simulink model "optical_flow_sim"  (R2024b)
settings: Solver=VariableStepAuto  StartTime=0.0  StopTime=30  RelTol=1e-3
undefined symbols (not defined in the file or in its folder): twist
libraries: ros2lib x4
settings Model: Creator=DCHOME  LastModifiedBy=DCHOME

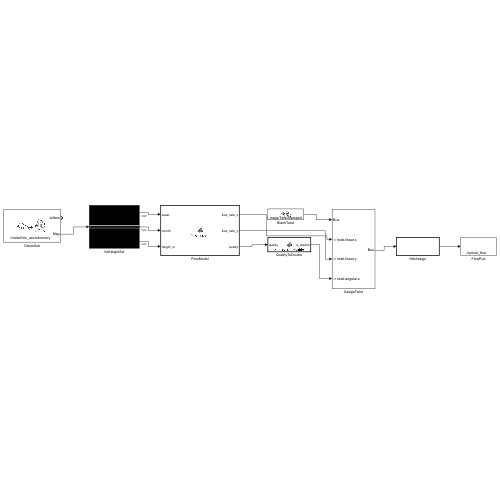
[thumbnail: Simulink's stored preview of the top-level diagram]
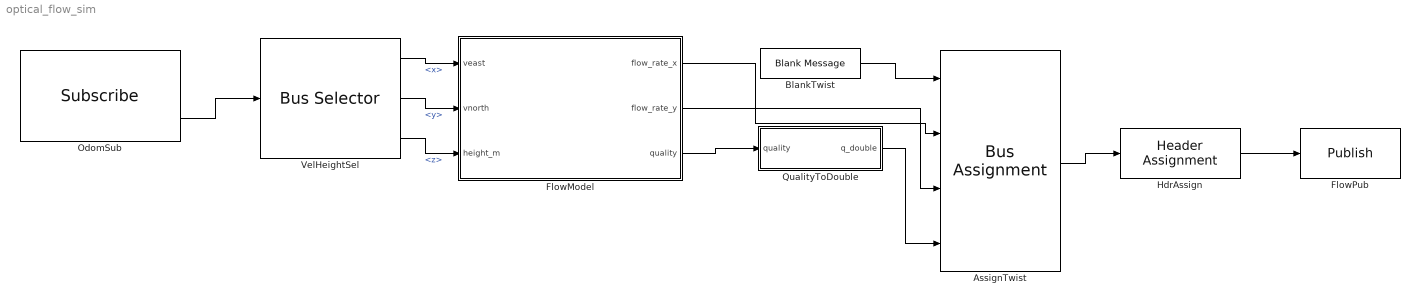
== system optical_flow_sim ==
  AssignTwist : BusAssignment  AssignedSignals=twist.linear.x,twist.linear.y,twist.angular.z
  BlankTwist : ros2lib/Blank Message  messageClass=Message  entityType=geometry_msgs/TwistStamped  messageType=geometry_msgs/TwistStamped  SampleTime=inf
  FlowModel : MATLAB Function  TreatAsAtomicUnit=on
  FlowPub : ros2lib/Publish  topicSource=Specify your own  topic=/optical_flow  messageType=geometry_msgs/TwistStamped  QOSHistory=Keep last  QOSDepth=1  QOSReliability=Reliable  QOSDurability=Volatile  QOSDeadline=Inf  QOSLifespan=Inf  QOSLiveliness=Automatic  QOSLeaseDuration=Inf  QOSAvoidROSNamespaceConventions=off
  HdrAssign : ros2lib/Header Assignment  SetFrameID=on  FrameID=optical_flow  InsertTimeStamp=on  SetHeaderFieldName=Use the default header field name  HeaderFieldName=header
  OdomSub : ros2lib/Subscribe  topicSource=Specify your own  topic=/model/iris_uav/odometry  messageType=nav_msgs/Odometry  sampleTime=0.05  QOSHistory=Keep last  QOSDepth=1  QOSReliability=Reliable  QOSDurability=Volatile  QOSDeadline=Inf  QOSLifespan=Inf  QOSLiveliness=Automatic  QOSLeaseDuration=Inf  QOSAvoidROSNamespaceConventions=off
  QualityToDouble : MATLAB Function  TreatAsAtomicUnit=on
  VelHeightSel : BusSelector  OutputSignals=twist.twist.linear.x,twist.twist.linear.y,pose.pose.position.z
  wires:
  OdomSub/2 -> VelHeightSel/1
  VelHeightSel/1 -> FlowModel/1(veast)  "<x>"
  VelHeightSel/2 -> FlowModel/2(vnorth)  "<y>"
  VelHeightSel/3 -> FlowModel/3(height_m)  "<z>"
  FlowModel/3(quality) -> QualityToDouble/1(quality)
  BlankTwist/1 -> AssignTwist/1
  FlowModel/1(flow_rate_x) -> AssignTwist/2
  FlowModel/2(flow_rate_y) -> AssignTwist/3
  QualityToDouble/1(q_double) -> AssignTwist/4
  AssignTwist/1 -> HdrAssign/1
  HdrAssign/1 -> FlowPub/1

== matlab function optical_flow_sim/QualityToDouble ==
  data: quality input; q_double output
function q_double = quality_to_double(quality)
    q_double = double(quality);
end

== matlab function optical_flow_sim/FlowModel ==
  data: veast input; flow_rate_x output; vnorth input; height_m input; flow_rate_y output; quality output
function [flow_rate_x, flow_rate_y, quality] = flow_model(veast, vnorth, height_m)
    FLOW_OPTIMAL_HEIGHT_M = 3.0000;
    FLOW_MIN_USABLE_HEIGHT_M = 0.3000;
    FLOW_MAX_USABLE_HEIGHT_M = 15.0000;
    WATER_QUALITY_FACTOR = 0.5500;
    NOISE_STDDEV_FRAC = 0.0500;
    h = max(height_m, 0.05); % avoid divide-by-zero right at the surface
    true_rate_x = -veast / h;  % small-angle optical-flow approximation
    true_rate_y =  vnorth / h;
    flow_rate_x = true_rate_x + NOISE_STDDEV_FRAC * abs(true_rate_x) * randn();
    flow_rate_y = true_rate_y + NOISE_STDDEV_FRAC * abs(true_rate_y) * randn();
    if h < FLOW_MIN_USABLE_HEIGHT_M || h > FLOW_MAX_USABLE_HEIGHT_M
        quality = uint8(0);
    else
        % U-shaped altitude quality curve, peak at FLOW_OPTIMAL_HEIGHT_M,
        % scaled down by the ambient open-water penalty.
        dist_from_optimal = abs(h - FLOW_OPTIMAL_HEIGHT_M) / FLOW_OPTIMAL_HEIGHT_M;
        base_q = max(0, 1 - 0.5 * dist_from_optimal);
        q = base_q * WATER_QUALITY_FACTOR * 255;
        quality = uint8(max(0, min(255, round(q + randn() * 10))));
    end
end
